simulink model "DC_MOTOR_pwm"  (R2018a)
settings: Solver=VariableStepAuto  StartTime=0.0  StopTime=80  RelTol=1e-3
model workspace (MAT data in the model file):
  B = 2.21978586253e-20
  J = 0.000193943815709
  K = 0.0137802290227
  L = 0.133562051134
  R = 0.505694900414
libraries: simulink_extras x2
settings Model: Creator=Hazem Elwakeel  LastModifiedBy=Hazem Elwakeel

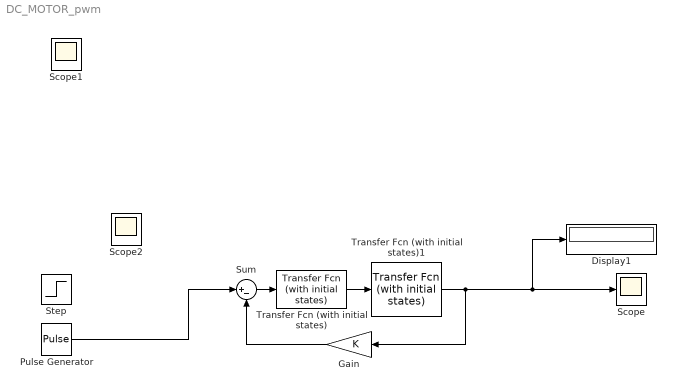
== system DC_MOTOR_pwm ==
  Display1 : Display
  Gain : Gain  Gain=K
  Pulse Generator : DiscretePulseGenerator  PulseType=Time based  Amplitude=1023  Period=20  PulseWidth=50
  Scope : Scope
  Scope2 : Scope
  Step : Step  After=1023  SampleTime=0.5
  Sum : Sum  Inputs=|+-
  Transfer Fcn (with initial states) : simulink_extras/Additional Linear/Transfer Fcn (with initial states)  N=[K]  D="[J  B]"  X0=.5
  Transfer Fcn (with initial states)1 : simulink_extras/Additional Linear/Transfer Fcn (with initial states)  N=[1]  D="[L  R]"  X0=.5
  Scope1 : Scope
  wires:
  Transfer Fcn (with initial states)/1 -> Transfer Fcn (with initial states)1/1
  Sum/1 -> Transfer Fcn (with initial states)/1
  Gain/1 -> Sum/2
  Transfer Fcn (with initial states)1/1 -> Scope/1, Display1/1, Gain/1
  Pulse Generator/1 -> Sum/1
